simulink model "puma560withSineInput"  (R2014a)
settings: Solver=ode3  StartTime=0.0  StopTime=inf  FixedStep=0.1  RelTol=1e-3
undefined symbols (not defined in the file): B, J, Ki, Km, Kp
libraries: roblocks x5, simulink x1
settings Model: ExtModeTrigMode=oneshot  ExtModeArmWhenConnect=off  ExtModeAutoUpdateStatusClock=off  Creator=pic  LastModifiedBy=Flavio
settings DataIOCC: LimitDataPoints=off  SignalLoggingSaveFormat=ModelDataLogs  SignalLoggingName=sigsOut
settings OptimizationCC: BlockReduction=off  BooleanDataType=off  ExpressionDepthLimit=2147483647
settings DebuggingCC: SaveWithParameterizedLinksMsg=none  UnderspecifiedInitializationDetection=Classic  SignalResolutionControl=TryResolveAllWithWarning  SolverPrmCheckMsg=none  MultiTaskDSMMsg=warning  MultiTaskCondExecSysMsg=none  FcnCallInpInsideContextMsg=UseLocalSettings  StateNameClashWarn=warning
settings HardwareCC: TargetUnknown=on
settings RTWCC: IncludeERTFirstTime=on
settings GRTTargetCC: CombineOutputUpdateFcns=off  GRTInterface=on

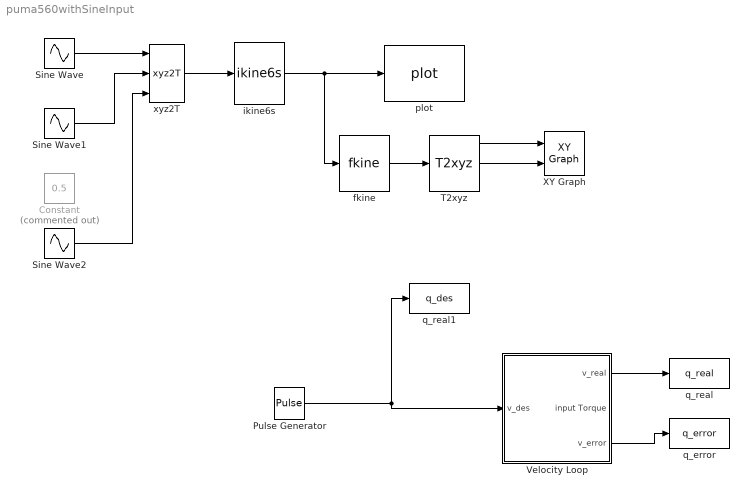
== system puma560withSineInput ==
  Constant : Constant  Commented=on  Value=0.5
  Pulse Generator : DiscretePulseGenerator  PulseType=Time based  Amplitude=5  Period=5  PulseWidth=5
  Sine Wave : Sin  Amplitude=0.5  Frequency=0.1  SampleTime=0
  Sine Wave1 : Sin  Amplitude=0.5  Frequency=0.1  Phase=pi/2  SampleTime=0
  Sine Wave2 : Sin  Amplitude=0.1  Bias=0.3  Frequency=0.2  SampleTime=0
  T2xyz : roblocks/Transform Conversion/T2xyz
  Velocity Loop : Subsystem
  XY Graph : simulink/Sinks/XY Graph  xmin=-1  xmax=1  ymin=-1  ymax=1  st=-1
  fkine : roblocks/Kinematics/fkine  robot=p560
  ikine6s : roblocks/Kinematics/ikine6s  robot=p560  conf='luf'
  plot : roblocks/Robot Graphics/plot  robot=p560  fps=25  holdplot=on
  q_error : ToWorkspace  VariableName=q_error  SampleTime=-1
  q_real : ToWorkspace  VariableName=q_real  SampleTime=-1
  q_real1 : ToWorkspace  VariableName=q_des  SampleTime=-1
  xyz2T : roblocks/Transform Conversion/xyz2T
  wires:
  ikine6s/1 -> plot/1, fkine/1
  fkine/1 -> T2xyz/1
  T2xyz/1 -> XY Graph/1
  T2xyz/2 -> XY Graph/2
  xyz2T/1 -> ikine6s/1
  Sine Wave/1 -> xyz2T/1
  Sine Wave1/1 -> xyz2T/2
  Sine Wave2/1 -> xyz2T/3
  Pulse Generator/1 -> q_real1/1, Velocity Loop/1(v_des)
  Velocity Loop/3(v_error) -> q_error/1
  Velocity Loop/1(v_real) -> q_real/1

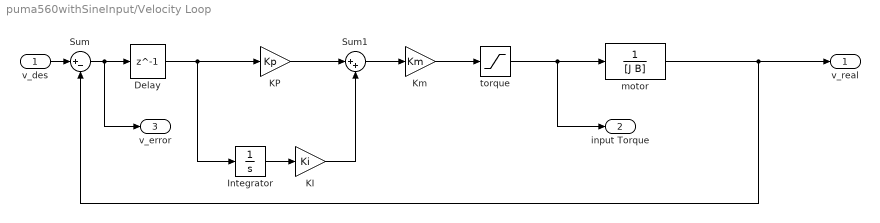
== system puma560withSineInput/Velocity Loop ==
  v_des : Inport
  Delay : Delay  DelayLength=1  InitialCondition=0  SampleTime=0.001
  Integrator : Integrator
  KI : Gain  Gain=Ki
  KP : Gain  Gain=Kp
  Km : Gain  Gain=Km
  Sum : Sum  Inputs=|+-
  Sum1 : Sum  Inputs=|++
  motor : TransferFcn  Denominator=[J B]
  torque : Saturate  UpperLimit=0.9  LowerLimit=-0.9
  v_real : Outport
  input Torque : Outport  Port=2
  v_error : Outport  Port=3
  wires:
  torque/1 -> input Torque/1, motor/1
  v_des/1 -> Sum/1
  motor/1 -> v_real/1, Sum/2
  KP/1 -> Sum1/1
  Delay/1 -> Integrator/1, KP/1
  Km/1 -> torque/1
  Sum/1 -> v_error/1, Delay/1
  Sum1/1 -> Km/1
  KI/1 -> Sum1/2
  Integrator/1 -> KI/1
